simulink model "Augmented"  (R2024a)
settings: Solver=VariableStepAuto  StartTime=0.0  StopTime=10.0  RelTol=1e-3
settings Model: Creator=bojack  LastModifiedBy=bojack

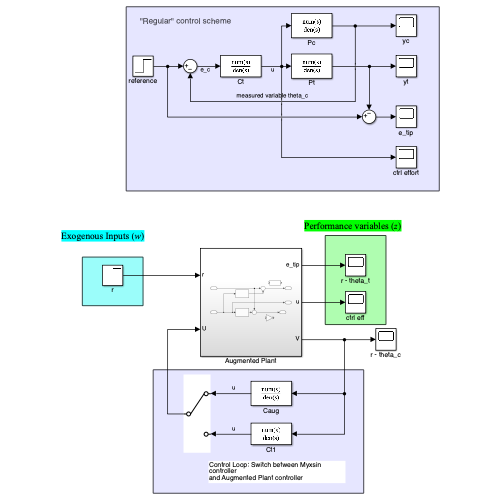
[thumbnail: Simulink's stored preview of the top-level diagram]
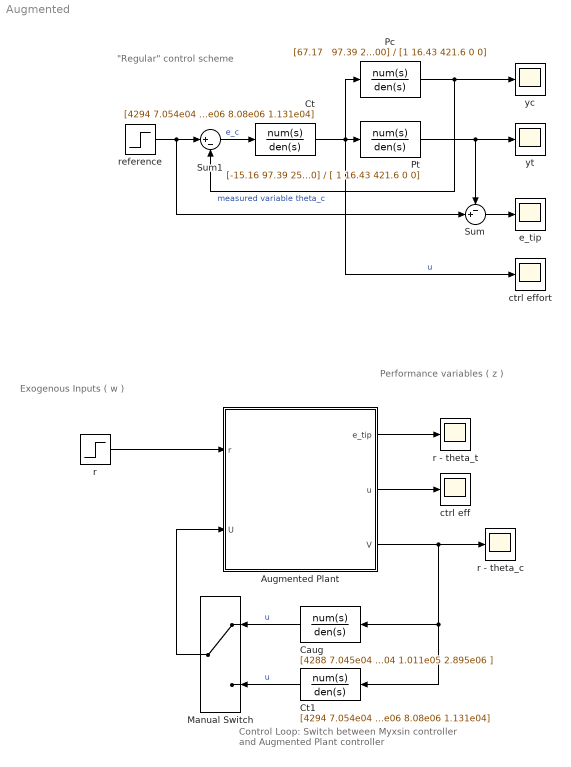
== system Augmented ==
  note: Control Loop: Switch between Myxsin controller
      | and Augmented Plant controller
  note: Performance variables ( z )
  note: "Regular" control scheme
  note: Exogenous Inputs ( w )
  Augmented Plant : Subsystem
  Caug : TransferFcn  Numerator=[4288 7.045e04 1.808e06 4895]  Denominator=|
      | [1 530.6 1.615e04 1.011e05 2.895e06
      | ]
  Ct : TransferFcn  Numerator=[4294 7.054e04 1.81e06 87.56 0.002116]  Denominator=[1 848.1 3.235e04 1.103e06 8.08e06 1.131e04]
  Ct1 : TransferFcn  Numerator=[4294 7.054e04 1.81e06 87.56 0.002116]  Denominator=[1 848.1 3.235e04 1.103e06 8.08e06 1.131e04]
  Manual Switch : ManualSwitch
  Pc : TransferFcn  Numerator="[67.17   97.39 2500]"  Denominator=[1 16.43 421.6 0 0]
  Pt : TransferFcn  Numerator=[-15.16 97.39 2500]  Denominator=[ 1 16.43 421.6 0 0]
  Sum : Sum  Inputs=-+|
  Sum1 : Sum  Inputs=|+-
  ctrl eff : Scope
  ctrl effort : Scope
  e_tip : Scope
  r : Step  Time=0  SampleTime=0
  r - theta_c : Scope
  r - theta_t : Scope
  reference : Step  Time=0  SampleTime=0
  yc : Scope
  yt : Scope
  wires:
  Sum1/1 -> Ct/1  "e_c"
  reference/1 -> Sum1/1, Sum/2
  Pc/1 -> yc/1, Sum1/2  "measured variable theta_c"
  Pt/1 -> Sum/1, yt/1
  Ct/1 -> Pc/1, Pt/1, ctrl effort/1  "u"
  Sum/1 -> e_tip/1
  r/1 -> Augmented Plant/1(r)
  Augmented Plant/1(e_tip) -> r - theta_t/1
  Augmented Plant/3(" V") -> r - theta_c/1, Caug/1, Ct1/1
  Augmented Plant/2(u) -> ctrl eff/1
  Ct1/1 -> Manual Switch/2  "u"
  Caug/1 -> Manual Switch/1  "u"
  Manual Switch/1 -> Augmented Plant/2(U)

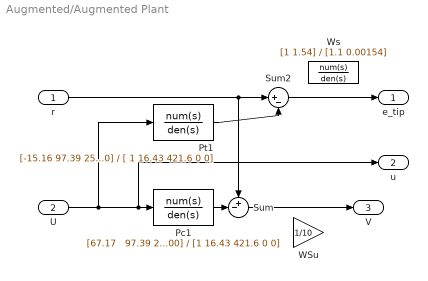
== system Augmented/Augmented Plant ==
  r : Inport
  U : Inport  Port=2
  Pc1 : TransferFcn  Numerator="[67.17   97.39 2500]"  Denominator=[1 16.43 421.6 0 0]
  Pt1 : TransferFcn  Numerator=[-15.16 97.39 2500]  Denominator=[ 1 16.43 421.6 0 0]
  Sum : Sum  Inputs=+-|
  Sum2 : Sum  Inputs=|+-
  WSu : Gain  Gain=1/10
  Ws : TransferFcn  Numerator=[1 1.54]  Denominator=[1.1 0.00154]
  e_tip : Outport
  u : Outport  Port=2
  " V" : Outport  Port=3
  wires:
  U/1 -> u/1, Pc1/1, Pt1/1
  r/1 -> Sum2/1, Sum/1
  Pt1/1 -> Sum2/2
  Pc1/1 -> Sum/2
  Sum/1 -> " V"/1
  Sum2/1 -> e_tip/1
